simulink model "dcpController_ExperimentalPosVel"  (R2016b)
settings: Solver=ode5  StartTime=0.0  StopTime=inf  FixedStep=0.001  RelTol=1e-3  EnableMultiTasking=on
undefined symbols (not defined in the file): robot, Standard_Devices, UDP_Protocol
libraries: dcpctrl x20, simulink x6, kukaslxctrl x1, sldrtlib x1
(part 2 of 2)

== system dcpController_ExperimentalPosVel/qraw2qjoint_filter/qrawcompfilt_J3 ==
  qraw_J3 : Inport
  Complementary Filter : dcpctrl/complementaryFilter
  Demux1 : Demux  Outputs=2
  Equal Moving Average : DiscreteFir  Coefficients=repmat([1/50],1,50)  InputProcessing=Columns as channels (frame based)
  Mux1 : Mux  Inputs=3
  compFiltTau_J4 : Constant  Value=0.036
  qraw2q_J3 : dcpctrl/qraw2q_J3
  q_J3 : Outport
  qd_J3 : Outport  Port=2
  wires:
  Equal Moving Average/1 -> qd_J3/1
  qraw_J3/1 -> qraw2q_J3/1
  Demux1/2 -> Complementary Filter/2, Mux1/1
  Demux1/1 -> Mux1/2
  qraw2q_J3/2 -> Complementary Filter/1, Equal Moving Average/1
  compFiltTau_J4/1 -> Complementary Filter/3
  qraw2q_J3/1 -> Demux1/1
  Complementary Filter/1 -> q_J3/1

== system dcpController_ExperimentalPosVel/qraw2qjoint_filter/qrawcompfilt_J4 ==
  qraw_J4 : Inport
  Complementary Filter : dcpctrl/complementaryFilter
  Demux1 : Demux  Outputs=2
  Equal Moving Average : DiscreteFir  Coefficients=repmat([1/50],1,50)  InputProcessing=Columns as channels (frame based)
  Mux1 : Mux  Inputs=3
  compFiltTau_J4 : Constant  Value=0.036
  qraw2q_J4 : dcpctrl/qraw2q_J4
  q_J4 : Outport
  qd_J4 : Outport  Port=2
  wires:
  qraw2q_J4/1 -> Demux1/1
  compFiltTau_J4/1 -> Complementary Filter/3
  qraw2q_J4/2 -> Equal Moving Average/1, Complementary Filter/1
  Demux1/1 -> Mux1/2
  Demux1/2 -> Mux1/1, Complementary Filter/2
  qraw_J4/1 -> qraw2q_J4/1
  Equal Moving Average/1 -> qd_J4/1
  Complementary Filter/1 -> Mux1/3, q_J4/1

== system dcpController_ExperimentalPosVel/AT40GW_PFFCtrl1/qdraw2pwm/qdraw2pwm_J1 ==
  qdraw_J1 : Inport
  Lookup Table Dynamic_J1 : simulink/Lookup Tables/Lookup Table Dynamic  LookUpMeth=Interpolation-Use End Values  OutDataType=fixdt('double')  OutScaling=[]  OutputDataTypeScalingMode=Specify via dialog  OutDataTypeStr=fixdt('double')  DoSatur=off
  pwm : FromWorkspace  VariableName=robot.J1qdr2PWMmap(:,1)'  SampleTime=0
  qdr : FromWorkspace  VariableName=robot.J1qdr2PWMmap(:,2)'  SampleTime=0
  pwm_J1 : Outport
  wires:
  pwm/1 -> Lookup Table Dynamic_J1/3
  qdr/1 -> Lookup Table Dynamic_J1/2
  qdraw_J1/1 -> Lookup Table Dynamic_J1/1
  Lookup Table Dynamic_J1/1 -> pwm_J1/1

== system dcpController_ExperimentalPosVel/AT40GW_PFFCtrl1/qdraw2pwm/qdraw2pwm_J2 ==
  qdraw_J2 : Inport
  Lookup Table Dynamic_J2 : simulink/Lookup Tables/Lookup Table Dynamic  LookUpMeth=Interpolation-Use End Values  OutDataType=fixdt('double')  OutScaling=[]  OutputDataTypeScalingMode=Specify via dialog  OutDataTypeStr=fixdt('double')  DoSatur=off
  pwm : FromWorkspace  VariableName=robot.J2qdr2PWMmap(:,1)'  SampleTime=0
  qdraw : FromWorkspace  VariableName=robot.J2qdr2PWMmap(:,2)'  SampleTime=0
  pwm_J2 : Outport
  wires:
  pwm/1 -> Lookup Table Dynamic_J2/3
  qdraw/1 -> Lookup Table Dynamic_J2/2
  qdraw_J2/1 -> Lookup Table Dynamic_J2/1
  Lookup Table Dynamic_J2/1 -> pwm_J2/1

== system dcpController_ExperimentalPosVel/AT40GW_PFFCtrl1/qdraw2pwm/qdraw2pwm_J3 ==
  qdraw_J3 : Inport
  Lookup Table DynamicJ3 : simulink/Lookup Tables/Lookup Table Dynamic  LookUpMeth=Interpolation-Use End Values  OutDataType=fixdt('double')  OutScaling=[]  OutputDataTypeScalingMode=Specify via dialog  OutDataTypeStr=fixdt('double')  DoSatur=off
  pwm : FromWorkspace  VariableName=robot.J3qdr2PWMmap(:,1)'  SampleTime=0
  qdraw : FromWorkspace  VariableName=robot.J3qdr2PWMmap(:,2)'  SampleTime=0
  pwm_J3 : Outport
  wires:
  pwm/1 -> Lookup Table DynamicJ3/3
  qdraw/1 -> Lookup Table DynamicJ3/2
  qdraw_J3/1 -> Lookup Table DynamicJ3/1
  Lookup Table DynamicJ3/1 -> pwm_J3/1

== system dcpController_ExperimentalPosVel/AT40GW_PFFCtrl1/qdraw2pwm/qdraw2pwm_J4 ==
  qdraw_J4 : Inport
  Lookup Table Dynamic_J4 : simulink/Lookup Tables/Lookup Table Dynamic  LookUpMeth=Interpolation-Use End Values  OutDataType=fixdt('double')  OutScaling=[]  OutputDataTypeScalingMode=Specify via dialog  OutDataTypeStr=fixdt('double')  DoSatur=off
  pwm : FromWorkspace  VariableName=robot.J4qdr2PWMmap(:,1)'  SampleTime=0
  qdraw : FromWorkspace  VariableName=robot.J4qdr2PWMmap(:,2)'  SampleTime=0
  pwm_J4 : Outport
  wires:
  pwm/1 -> Lookup Table Dynamic_J4/3
  qdraw/1 -> Lookup Table Dynamic_J4/2
  qdraw_J4/1 -> Lookup Table Dynamic_J4/1
  Lookup Table Dynamic_J4/1 -> pwm_J4/1

== system dcpController_ExperimentalPosVel/qraw2qjoint_filter/J1 Conversion & Comp Filtering/Slider ==

== matlab function dcpController_ExperimentalPosVel/AT40GW_PFFCtrl1/qd2qdraw/dj2drfcn ==
  data: q input; qdraw output; qd input
function qdraw = fcn(q,qd)
%#codegen

qdraw = dj2drfcn_at40gw(q(2),q(3))*qd;

== matlab function dcpController_ExperimentalPosVel/Cartesian Position Vizualization/fkine_at40gw ==
  data: q input; x output
function x = fcn(q)
%#codegen

x_temp = fkine_at40gw(q(1),q(2),q(3),q(4))*[1;0;0;0];
x = x_temp(2:4);

== matlab function dcpController_ExperimentalPosVel/LIFXcontrol/Hue Changer ==
  data: h input; y output size=[1,49]; s input; b input; k input
function y = fcn(h,s,b,k)
%#codegen
%%
dec_code = [49;0;0;52;0;0;0;0;0;0;0;0;0;0;0;0;0;0;0;0;0;0;0;0;0;0;0;0;0;0;0;0;102;0;0;0;0;85;85;255;255;255;255;191;218;0;0;0;0];
%%
%%HUE 
hue = h/360 * 65535; %hue conversion formula, from degrees scale to LIFX scale
hue = floor(hue);
hue_hex = dec2hex(hue);

if (length(hue_hex) == 1)
    hue_arr = ['0',hue_hex(1)];
    hue_arr = ['00',hue_arr(1:2)];

elseif (length(hue_hex) ==2)
    hue_arr = ['00',hue_hex(1:2)];  
    
elseif (length(hue_hex) == 3)
    hue_arr = ['0', hue_hex(1), hue_hex(2), hue_hex(3)];
    hue_arr = [hue_arr(1:2),hue_arr(3:4)];
    
else
    hue_arr = [hue_hex(1:2), hue_hex(3:4)];
        
end

hue_out = hex2dec(hue_arr(1:2));
hue_out2 = hex2dec(hue_arr(3:4));

dec_code(38) = hue_out2;
dec_code(39) = hue_out;

%%
%SATURATION
sat = s * 65535; %saturation conversion formula, from 0-1 to LIFX scale
sat = floor(sat);
sat_hex = dec2hex(sat);

if (length(sat_hex) == 1)
    sat_arr = ['0',sat_hex(1)];
    sat_arr = ['00',sat_arr(1:2)];

elseif (length(sat_hex) ==2)
    sat_arr = ['00',sat_hex(1:2)];  
    
elseif (length(sat_hex) == 3)
    sat_arr = ['0', sat_hex(1), sat_hex(2), sat_hex(3)];
    sat_arr = [sat_arr(1:2),sat_arr(3:4)];
    
else
    sat_arr = [sat_hex(1:2), sat_hex(3:4)];
        
end

sat_out = hex2dec(sat_arr(1:2));
sat_out2 = hex2dec(sat_arr(3:4));

dec_code(40) = sat_out2;
dec_code(41) = sat_out;

%%

%BRIGHTNESS
bright = b * 65535; %brightness conversion formula, from 0-1 to LIFX scale
bright = floor(bright);
bright_hex = dec2hex(bright);

if (length(bright_hex) == 1)
    bright_arr = ['0',bright_hex(1)];
    bright_arr = ['00',bright_arr(1:2)];

elseif (length(bright_hex) ==2)
    bright_arr = ['00',bright_hex(1:2)];  
    
elseif (length(bright_hex) == 3)
    bright_arr = ['0', bright_hex(1), bright_hex(2), bright_hex(3)];
    bright_arr = [bright_arr(1:2),bright_arr(3:4)];
    
else
    bright_arr = [bright_hex(1:2), bright_hex(3:4)];
end

bright_out = hex2dec(bright_arr(1:2));
bright_out2 = hex2dec(bright_arr(3:4));

dec_code(42) = bright_out2;
dec_code(43) = bright_out;

%%
%KELVIN
kelvin = k; %Kelvin conversion formula, from 0-1 to LIFX scale
kelvin = floor(kelvin);
kelvin_hex = dec2hex(kelvin);

if (length(kelvin_hex) == 1)
    kelvin_arr = ['0',kelvin_hex(1)];
    kelvin_arr = ['00',kelvin_arr(1:2)];

elseif (length(kelvin_hex) ==2)
    kelvin_arr = ['00',kelvin_hex(1:2)];  
    
elseif (length(kelvin_hex) == 3)
    kelvin_arr = ['0', kelvin_hex(1), kelvin_hex(2), kelvin_hex(3)];
    kelvin_arr = [kelvin_arr(1:2), kelvin_arr(3:4)];
    
else
    kelvin_arr = [kelvin_hex(1:2), kelvin_hex(3:4)];
end

kelvin_out = hex2dec(kelvin_arr(1:2));
kelvin_out2 = hex2dec(kelvin_arr(3:4));

dec_code(44) = kelvin_out2;
dec_code(45) = kelvin_out;

%%
%y_temp = char_out;
%y = y_temp(1:2);

y = uint8(dec_code');
